simulink model "Two_Channel_FP_Teleoperation"  (R2022b)
settings: Solver=VariableStepAuto  StartTime=0.0  StopTime=15  RelTol=1e-3
values from neighbouring files (symbols this model uses):
  alpha = 1    [parameters.m]
  Amp = 15    [parameters.m]    (also in parameters_kalman.m)
  Be = 100    [parameters.m]    (also in parameters_kalman.m)
  beta = 0.1    [parameters.m]
  Bh = 1    [parameters.m]    (also in parameters_kalman.m)
  Bm = 20*0.8    (= 16)    [parameters.m]    (also in parameters_kalman.m)
  Bs = 4*Bm    (= 64)    [parameters.m]    (also in parameters_kalman.m)
  delay = 10    [parameters.m]    (also in parameters_kalman.m)
  Dh = 20*0.8    (= 16)    [parameters.m]    (also in parameters_kalman.m)
  Dm = 1.3    [parameters.m]    (also in parameters_kalman.m = 5.3)
  Ds = 1.2    [parameters.m]    (also in parameters_kalman.m)
  Fc = 1    [parameters.m]    (also in parameters_kalman.m)
  Flp = 5    [parameters.m]    (also in parameters_kalman.m)
  Hd = 1000    [parameters.m]
  Hm_init = 0    [parameters.m]
  Hs_init = 0    [parameters.m]
  Jh = 1    [parameters.m]    (also in parameters_kalman.m)
  Ke = 200    [parameters.m]    (also in parameters_kalman.m)
  Km = 10*1    (= 10)    [parameters.m]    (also in parameters_kalman.m)
  Ks = 4*Km    (= 40)    [parameters.m]    (also in parameters_kalman.m)
  Mm = 0.5    [parameters.m]    (also in parameters_kalman.m)
  Ms = 2    [parameters.m]    (also in parameters_kalman.m)
  Ph = 10*1    (= 10)    [parameters.m]    (also in parameters_kalman.m)
  Ts = 0.001    [parameters.m]    (also in parameters_kalman.m)
  xe = 3    [parameters.m]    (also in parameters_kalman.m = 30)
undefined symbols (not defined in the file or in its folder): DiscIntNeverNeededParam
libraries: simulink x3
settings Model: Creator=uzair  LastModifiedBy=uzair

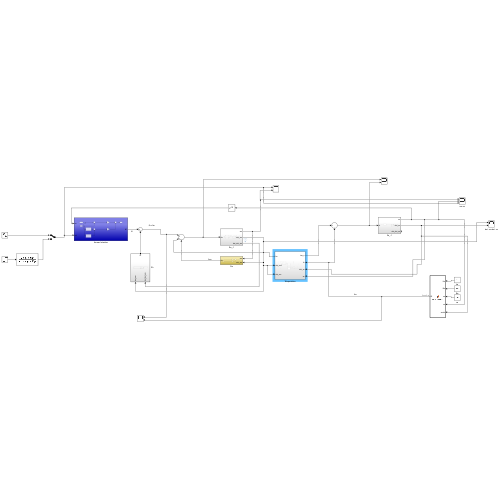
[thumbnail: Simulink's stored preview of the top-level diagram]
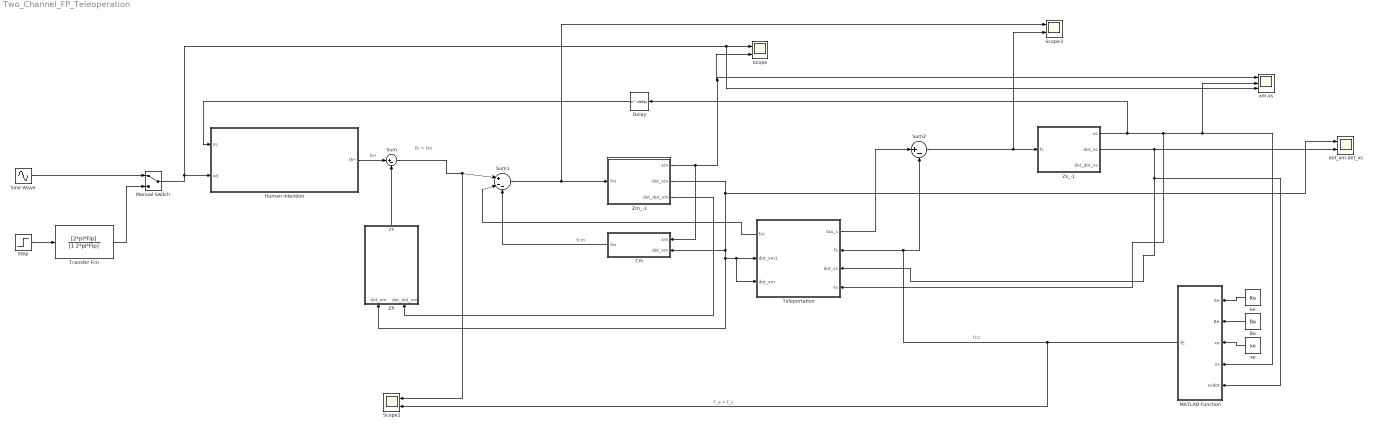
== system Two_Channel_FP_Teleoperation ==
  note: fcs
  note: fcm
  note: fh = fm
  Be : Constant  Value=Be
  Cm : Subsystem
  Delay : Delay  DelayLength=delay  SampleTime=Ts
  Human Intention : Subsystem
  MATLAB Function : MATLAB Function  TreatAsAtomicUnit=on
  Manual Switch : ManualSwitch
  Scope : Scope  NumInputPorts=2
  Scope2 : Scope  NumInputPorts=2
  Scope3 : Scope  NumInputPorts=2
  Sine Wave : Sin  Amplitude=Amp  Frequency=2*pi*Fc  SampleTime=Ts
  Step : Step  Time=0.5  After=Amp  SampleTime=Ts
  Sum : Sum  Inputs=|+-
  Sum1 : Sum  Inputs=|+--
  Sum2 : Sum  Inputs=|+-
  Teleportation : Subsystem
      settings: PortSchema="{\"entries\":[{\"content\":{\"sides\":[{\"content\":{\"connectorIds\":[\"Out2\",\"In1\",\"In2\"]},\"type\":\"ConnectorPlacement.EquallySpacedRectSide\",\"uuid\":\"b5f7abc7-c75d-4363-a17a-8f86c90608cd\"},{\"content\":{\"connectorIds\":[\"Out1\",\"In3\",\"In4\",\"In5\"],\"side\":\"RIGHT\"},\"type\":\"ConnectorPlacement.EquallySpacedRectSide\",\"uuid\":\"2ed87bee-e320-4c73-a1d3-1960a55b558d\"},{\"content\":{\"connectorIds\":[],\"side\":\"TOP\"},\"type\":\"ConnectorPlacement.EquallySpacedRectSide\",\"uuid\":\"65d6df07-20ed-40e6-978a-52c206d58fbe\"}]},\"type\":\"ConnectorPlacement.EquallySpacedConnector\",\"uuid\":\"b3d72d1f-cf16-401b-a692-293857f5cfdb\"}],\"packageUris\":[\"http://schema.mathworks.com/mf0/Connector/R2020b\"],\"version\":\"1.0\"}"
  Transfer Fcn : TransferFcn  Numerator=[2*pi*Flp]  Denominator=[1 2*pi*Flp]
  Zh : Subsystem
  Zm_-1 : Subsystem
  Zs_-1 : Subsystem
  dot_xm-dot_xs : Scope  NumInputPorts=2
  ke : Constant  Value=Ke
  xe : Constant  Value=xe
  xm-xs : Scope  NumInputPorts=3
  wires:
  Sine Wave/1 -> Manual Switch/1
  Step/1 -> Transfer Fcn/1
  Transfer Fcn/1 -> Manual Switch/2
  Manual Switch/1 -> xm-xs/3, Scope/1, Human Intention/2(xd)
  Human Intention/1(fh*) -> Sum/1  "fh*"
  Zh/1(Zh) -> Sum/2
  Sum/1 -> Scope2/1, Sum1/1
  Sum1/1 -> Scope3/1, Zm_-1/1(fm)
  Zm_-1/3(dot_dot_xm) -> Zh/2(dot_dot_xm)
  Sum2/1 -> Scope3/2, Zs_-1/1(fs)
  Zs_-1/2(dot_xs) -> dot_xm-dot_xs/2, MATLAB Function/5(xsdot), Teleportation/4(dot_xs)
  xe/1 -> MATLAB Function/3(xe)
  Be/1 -> MATLAB Function/2(Be)
  ke/1 -> MATLAB Function/1(Ke)
  MATLAB Function/1(fE) -> Scope2/2, Sum2/2, Teleportation/3(fs)  "f_e = f_s"
  Teleportation/1(tau_s) -> Sum2/1
  Zm_-1/2(dot_xm) -> Zh/1(dot_xm), Teleportation/2(dot_xm), Teleportation/1(dot_xm1), Cm/2(dot_xm), dot_xm-dot_xs/1
  Zm_-1/1(xm) -> Scope/2, xm-xs/1, Cm/1(xm)
  Zs_-1/1(xs) -> Delay/1, Teleportation/5(xs), xm-xs/2, MATLAB Function/4(xs)
  Delay/1 -> Human Intention/1(xs)
  Teleportation/2(fm) -> Sum1/2
  Cm/1(fm) -> Sum1/3

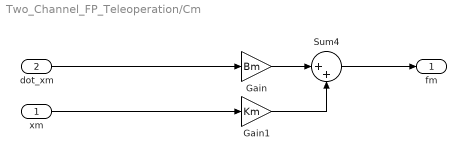
== system Two_Channel_FP_Teleoperation/Cm ==
  xm : Inport
  dot_xm : Inport  Port=2
  Gain : Gain  Gain=Bm
  Gain1 : Gain  Gain=Km
  Sum4 : Sum  Inputs=|++
  fm : Outport
  wires:
  Sum4/1 -> fm/1
  xm/1 -> Gain1/1
  Gain/1 -> Sum4/1
  Gain1/1 -> Sum4/2
  dot_xm/1 -> Gain/1

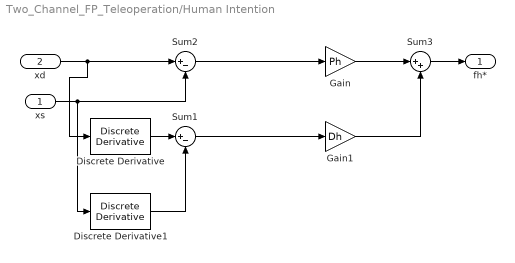
== system Two_Channel_FP_Teleoperation/Human Intention ==
  xs : Inport
  xd : Inport  Port=2
  Discrete Derivative : simulink/Discrete/Discrete Derivative  gainval=1.0  ICPrevScaledInput=0.0  OutMin=[]  OutMax=[]  OutDataType=fixdt(1, 16)  OutScaling=2^-10  DoSatur=off
  Discrete Derivative1 : simulink/Discrete/Discrete Derivative  gainval=1.0  ICPrevScaledInput=0.0  OutMin=[]  OutMax=[]  OutDataType=fixdt(1, 16)  OutScaling=2^-10  DoSatur=off
  Gain : Gain  Gain=Ph
  Gain1 : Gain  Gain=Dh
  Sum1 : Sum  Inputs=|+-
  Sum2 : Sum  Inputs=|+-
  Sum3 : Sum  Inputs=|++
  fh* : Outport
  wires:
  xs/1 -> Discrete Derivative1/1, Sum2/2
  Sum2/1 -> Gain/1
  Sum1/1 -> Gain1/1
  Gain1/1 -> Sum3/2
  Gain/1 -> Sum3/1
  xd/1 -> Discrete Derivative/1, Sum2/1
  Discrete Derivative/1 -> Sum1/1
  Discrete Derivative1/1 -> Sum1/2
  Sum3/1 -> fh*/1

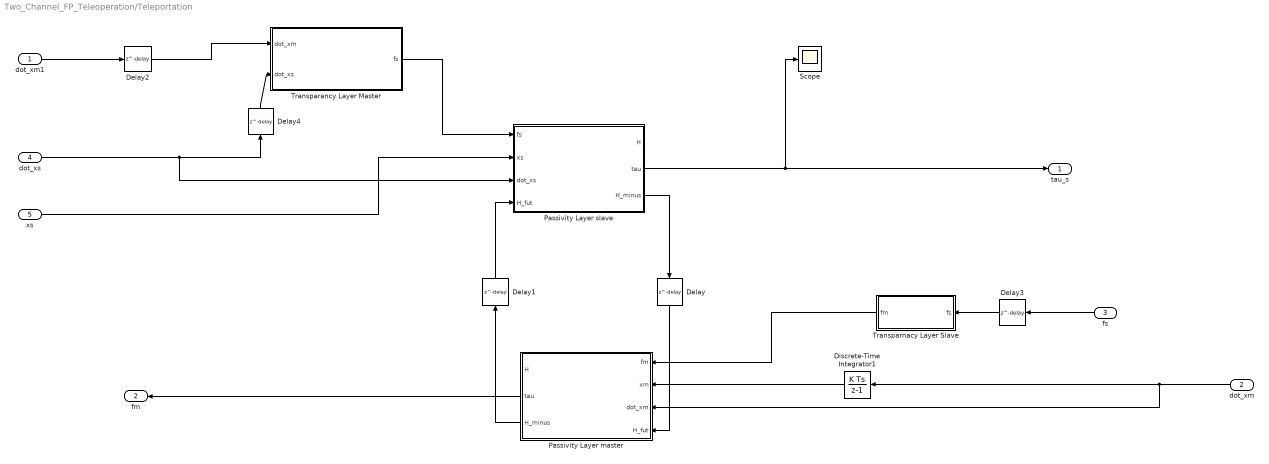
== system Two_Channel_FP_Teleoperation/Teleportation ==
  dot_xm1 : Inport
  dot_xm : Inport  Port=2
  fs : Inport  Port=3
  dot_xs : Inport  Port=4
  xs : Inport  Port=5
  Delay{,1..4} (5 alike) : Delay  DelayLength=delay
  Discrete-Time Integrator1 : DiscreteIntegrator  SampleTime=-1  ICPrevOutput=DiscIntNeverNeededParam  ICPrevScaledInput=DiscIntNeverNeededParam
  Passivity Layer master : MATLAB Function  TreatAsAtomicUnit=on
  Passivity Layer slave : MATLAB Function  TreatAsAtomicUnit=on
  Scope : Scope
  Transparancy Layer Master : Subsystem
  Transparnacy Layer Slave : Subsystem
  tau_s : Outport
  fm : Outport  Port=2
  wires:
  Passivity Layer master/2(tau) -> fm/1
  fs/1 -> Delay3/1
  Passivity Layer slave/2(tau) -> Scope/1, tau_s/1
  dot_xm/1 -> Passivity Layer master/3(dot_xm), Discrete-Time Integrator1/1
  Transparancy Layer Master/1(fs) -> Passivity Layer slave/1(fs)
  Transparnacy Layer Slave/1(fm) -> Passivity Layer master/1(fm)
  Passivity Layer slave/3(H_minus) -> Delay/1
  Passivity Layer master/3(H_minus) -> Delay1/1
  Discrete-Time Integrator1/1 -> Passivity Layer master/2(xm)
  Delay/1 -> Passivity Layer master/4(H_fut)
  Delay1/1 -> Passivity Layer slave/4(H_fut)
  Delay2/1 -> Transparancy Layer Master/1(dot_xm)
  Delay3/1 -> Transparnacy Layer Slave/1(fs)
  dot_xm1/1 -> Delay2/1
  dot_xs/1 -> Passivity Layer slave/3(dot_xs), Delay4/1
  xs/1 -> Passivity Layer slave/2(xs)
  Delay4/1 -> Transparancy Layer Master/2(dot_xs)

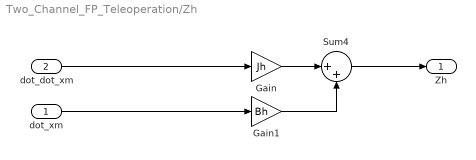
== system Two_Channel_FP_Teleoperation/Zh ==
  dot_xm : Inport
  dot_dot_xm : Inport  Port=2
  Gain : Gain  Gain=Jh
  Gain1 : Gain  Gain=Bh
  Sum4 : Sum  Inputs=|++
  Zh : Outport
  wires:
  dot_dot_xm/1 -> Gain/1
  Gain1/1 -> Sum4/2
  Gain/1 -> Sum4/1
  Sum4/1 -> Zh/1
  dot_xm/1 -> Gain1/1

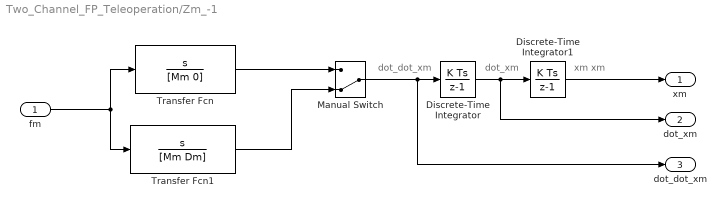
== system Two_Channel_FP_Teleoperation/Zm_-1 ==
  note: dot_dot_xm
  note: dot_xm
  note: xm
      | xm
  fm : Inport
  Discrete-Time Integrator : DiscreteIntegrator  SampleTime=Ts  ICPrevOutput=DiscIntNeverNeededParam  ICPrevScaledInput=DiscIntNeverNeededParam
  Discrete-Time Integrator1 : DiscreteIntegrator  SampleTime=Ts  ICPrevOutput=DiscIntNeverNeededParam  ICPrevScaledInput=DiscIntNeverNeededParam
  Manual Switch : ManualSwitch  CurrentSetting=0
  Transfer Fcn : TransferFcn  Numerator=[1 0]  Denominator=[Mm 0]
  Transfer Fcn1 : TransferFcn  Numerator=[1 0]  Denominator=[Mm Dm]
  xm : Outport
  dot_xm : Outport  Port=2
  dot_dot_xm : Outport  Port=3
  wires:
  Manual Switch/1 -> Discrete-Time Integrator/1, dot_dot_xm/1
  fm/1 -> Transfer Fcn/1, Transfer Fcn1/1
  Transfer Fcn/1 -> Manual Switch/1
  Transfer Fcn1/1 -> Manual Switch/2
  Discrete-Time Integrator1/1 -> xm/1
  Discrete-Time Integrator/1 -> dot_xm/1, Discrete-Time Integrator1/1

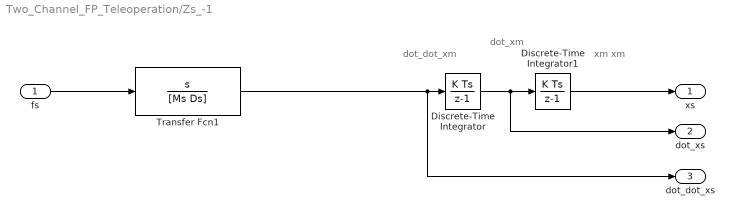
== system Two_Channel_FP_Teleoperation/Zs_-1 ==
  note: dot_dot_xm
  note: dot_xm
  note: xm
      | xm
  fs : Inport
  Discrete-Time Integrator : DiscreteIntegrator  SampleTime=Ts  ICPrevOutput=DiscIntNeverNeededParam  ICPrevScaledInput=DiscIntNeverNeededParam
  Discrete-Time Integrator1 : DiscreteIntegrator  SampleTime=Ts  ICPrevOutput=DiscIntNeverNeededParam  ICPrevScaledInput=DiscIntNeverNeededParam
  Transfer Fcn1 : TransferFcn  Numerator=[1 0]  Denominator=[Ms Ds]
  xs : Outport
  dot_xs : Outport  Port=2
  dot_dot_xs : Outport  Port=3
  wires:
  Transfer Fcn1/1 -> dot_dot_xs/1, Discrete-Time Integrator/1
  fs/1 -> Transfer Fcn1/1
  Discrete-Time Integrator/1 -> dot_xs/1, Discrete-Time Integrator1/1
  Discrete-Time Integrator1/1 -> xs/1

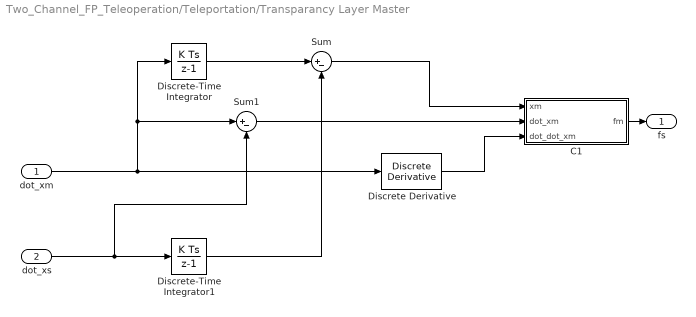
== system Two_Channel_FP_Teleoperation/Teleportation/Transparancy Layer Master ==
  dot_xm : Inport
  dot_xs : Inport  Port=2
  C1 : Subsystem
  Discrete Derivative : simulink/Discrete/Discrete Derivative  gainval=1.0  ICPrevScaledInput=0.0  OutMin=[]  OutMax=[]  OutDataType=fixdt(1, 16)  OutScaling=2^-10  DoSatur=off
  Discrete-Time Integrator : DiscreteIntegrator  SampleTime=Ts  ICPrevOutput=DiscIntNeverNeededParam  ICPrevScaledInput=DiscIntNeverNeededParam
  Discrete-Time Integrator1 : DiscreteIntegrator  SampleTime=Ts  ICPrevOutput=DiscIntNeverNeededParam  ICPrevScaledInput=DiscIntNeverNeededParam
  Sum : Sum  Inputs=|+-
  Sum1 : Sum  Inputs=|+-
  fs : Outport
  wires:
  dot_xm/1 -> Discrete Derivative/1, Sum1/1, Discrete-Time Integrator/1
  Discrete Derivative/1 -> C1/3(dot_dot_xm)
  C1/1(fm) -> fs/1
  dot_xs/1 -> Sum1/2, Discrete-Time Integrator1/1
  Discrete-Time Integrator/1 -> Sum/1
  Sum/1 -> C1/1(xm)
  Discrete-Time Integrator1/1 -> Sum/2
  Sum1/1 -> C1/2(dot_xm)

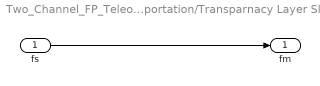
== system Two_Channel_FP_Teleoperation/Teleportation/Transparnacy Layer Slave ==
  fs : Inport
  fm : Outport
  wires:
  fs/1 -> fm/1

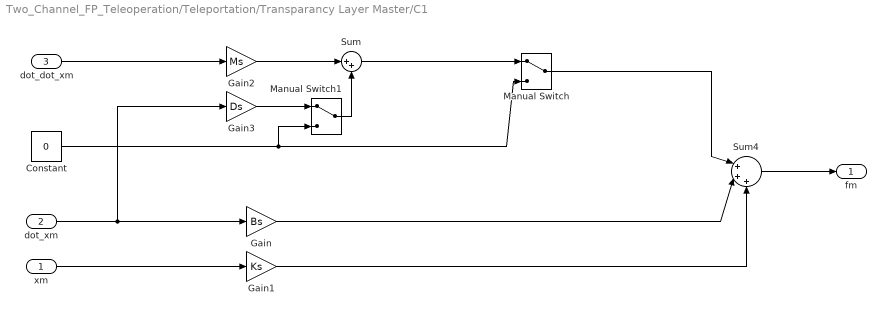
== system Two_Channel_FP_Teleoperation/Teleportation/Transparancy Layer Master/C1 ==
  xm : Inport
  dot_xm : Inport  Port=2
  dot_dot_xm : Inport  Port=3
  Constant : Constant  Value=0
  Gain : Gain  Gain=Bs
  Gain1 : Gain  Gain=Ks
  Gain2 : Gain  Gain=Ms
  Gain3 : Gain  Gain=Ds
  Manual Switch : ManualSwitch
  Manual Switch1 : ManualSwitch
  Sum : Sum  Inputs=|++
  Sum4 : Sum  Inputs=|+++
  fm : Outport
  wires:
  dot_xm/1 -> Gain3/1, Gain/1
  Gain/1 -> Sum4/2
  xm/1 -> Gain1/1
  Sum4/1 -> fm/1
  Gain1/1 -> Sum4/3
  Sum/1 -> Manual Switch/1
  Manual Switch/1 -> Sum4/1
  Constant/1 -> Manual Switch1/2, Manual Switch/2
  dot_dot_xm/1 -> Gain2/1
  Gain2/1 -> Sum/1
  Gain3/1 -> Manual Switch1/1
  Manual Switch1/1 -> Sum/2

== matlab function Two_Channel_FP_Teleoperation/Teleportation/Passivity Layer slave ==
  data: fs input; xs input; dot_xs input; H output; Hs_init parameter; H_fut input; Ts parameter; tau output; beta parameter; H_minus output
function [H, tau, H_minus] = fcn(fs,xs,dot_xs,Hs_init, H_fut, Ts, beta)
    persistent H_pre tau_pre xs_pre 

    if(isempty(H_pre))
        H_pre = Hs_init;
        tau_pre = 0;
        xs_pre = 0;
    end

    delta_H = tau_pre * (xs - xs_pre);
    H = H_pre + H_fut - delta_H;

    if(H <= 0)
        tau_max_1 = 0;
    else
        tau_max_1 = fs;
    end

    tau_max_2 = H/(dot_xs*Ts);

    tau = sign(fs)* min(abs(tau_max_1), abs(tau_max_2));

    H_minus = 0;
    if(H > 0)
        H_minus = beta*H;
        H = H - H_minus;
    end

    tau_pre = tau;
    xs_pre = xs;
    H_pre = H;
end

== matlab function Two_Channel_FP_Teleoperation/MATLAB Function ==
  data: Ke input; fE output; Be input; xe input; xs input; xsdot input
function fE = environment(Ke, Be, xe, xs, xsdot)
    if xs > xe
        fE = Ke * (xs - xe) + Be * xsdot; % Plot both contributions Ke and Be
    else
        fE = 0;
    end
end

== matlab function Two_Channel_FP_Teleoperation/Teleportation/Passivity Layer master ==
  data: fm input; xm input; dot_xm input; H output; Hm_init parameter; H_fut input; Ts parameter; tau output; beta parameter; H_minus output; Hd parameter; alpha parameter
function [H, tau, H_minus] = fcn(fm,xm,dot_xm,Hm_init, H_fut, Ts, beta, Hd, alpha)
    persistent H_pre tau_pre xm_pre 

    if(isempty(H_pre))
        H_pre = Hm_init;
        tau_pre = 0;
        xm_pre = 0;
    end

    delta_H = tau_pre * (xm - xm_pre);
    H = H_pre + H_fut - delta_H;

    if(H <= 0)
        tau_max_1 = 0;
    else
        tau_max_1 = fm;
    end

    if(abs(dot_xm) < 0.001)
        tau_max_2 = sign(dot_xm)*10000;
    else
        tau_max_2 = H/(dot_xm*Ts);
    end

    

   

    tau = sign(fm)* min(abs(tau_max_1), abs(tau_max_2));

    % Use tlc if necessary
    if(H < Hd)
       d = alpha*(Hd - H);
       tau_TLC = -1*d*dot_xm;
       tau = tau + tau_TLC;
    end

    H_minus = 0;
    if(H > 0)
        H_minus = beta*H;
        H = H - H_minus;
    end

    tau_pre = tau;
    xm_pre = xm;
    H_pre = H;
end
